simulink model "Q410_sim"  (R2021b)
settings: Solver=ode45  StartTime=0.0  StopTime=50  MinStep=0.0000001  RelTol=1e-3
values from neighbouring files (symbols this model uses):
  A = poly([-0.5 ,-3])    [Q410.m]
  A_m = [1 2*zeta*omega_n omega_n^2]    [Q410.m]
  alpha = .3    (= 0.3)    [Q410.m]
  B = 3    [Q410.m]
  P_0 = 1e12*eye(4)    [Q410.m]
  T = .0001    (= 0.0001)    [Q410.m]
settings Model: Creator=YSNsec  LastModifiedBy=YSNsec

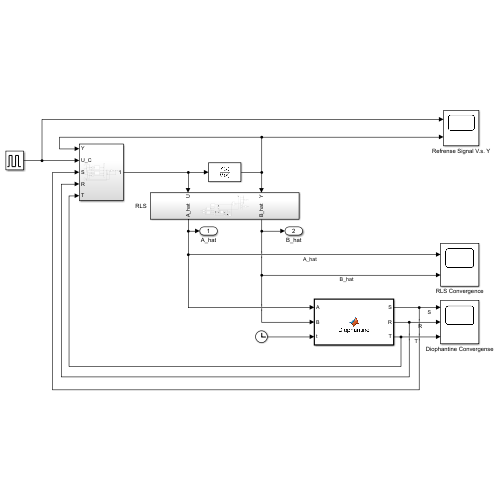
[thumbnail: Simulink's stored preview of the top-level diagram]
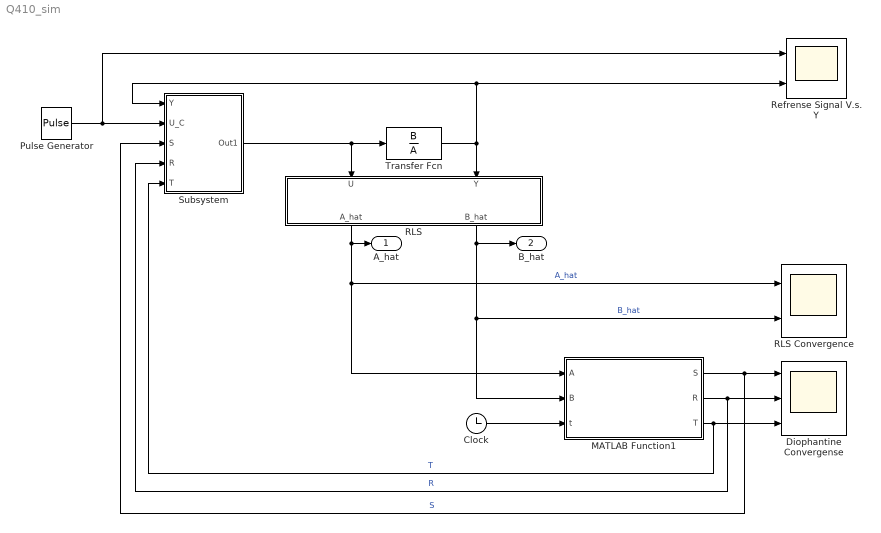
== system Q410_sim ==
  Clock : Clock
  Diophantine Convergense : Scope  NumInputPorts=3
  MATLAB Function1 : MATLAB Function  TreatAsAtomicUnit=on
  Pulse Generator : DiscretePulseGenerator  PulseType=Time based  Period=6  PulseWidth=50
  RLS : Subsystem
  RLS Convergence : Scope  NumInputPorts=2
  Refrense Signal V.s. Y : Scope  NumInputPorts=2
  Subsystem : Subsystem
  Transfer Fcn : TransferFcn  Numerator=B  Denominator=A
  A_hat : Outport  VectorParamsAs1DForOutWhenUnconnected=off
  B_hat : Outport  Port=2  VectorParamsAs1DForOutWhenUnconnected=off
  wires:
  Clock/1 -> MATLAB Function1/3(t)
  RLS/2(B_hat) -> B_hat/1, MATLAB Function1/2(B), RLS Convergence/2  "B_hat"
  RLS/1(A_hat) -> A_hat/1, RLS Convergence/1, MATLAB Function1/1(A)  "A_hat"
  MATLAB Function1/1(S) -> Diophantine Convergense/1, Subsystem/3(S)  "S"
  MATLAB Function1/2(R) -> Diophantine Convergense/2, Subsystem/4(R)  "R"
  MATLAB Function1/3(T) -> Diophantine Convergense/3, Subsystem/5(T)  "T"
  Transfer Fcn/1 -> Refrense Signal V.s. Y/2, Subsystem/1(Y), RLS/2(Y)
  Subsystem/1(Out1) -> Transfer Fcn/1, RLS/1(U)
  Pulse Generator/1 -> Subsystem/2(U_C), Refrense Signal V.s. Y/1

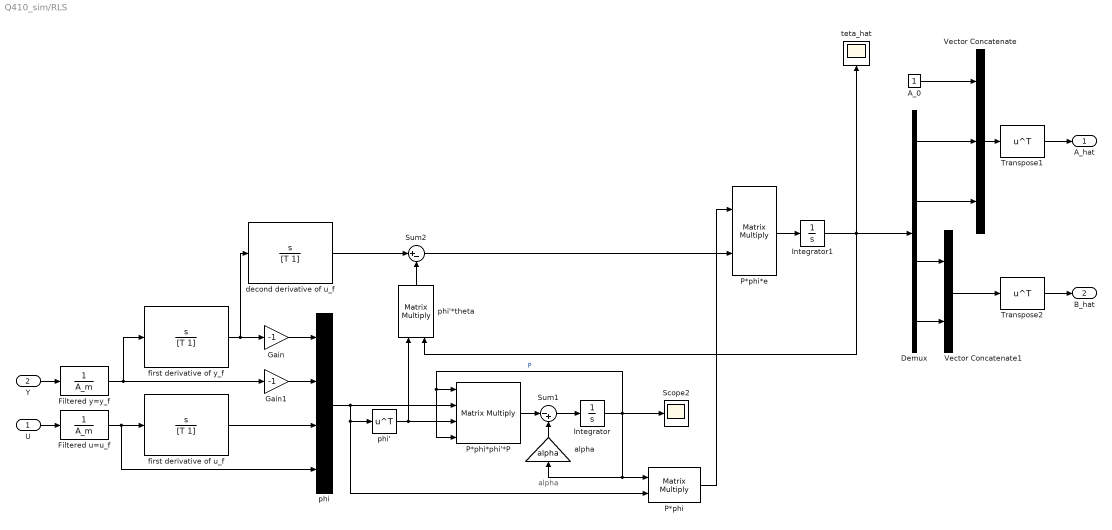
== system Q410_sim/RLS ==
  note: alpha
  U : Inport
  Y : Inport  Port=2
  A_0 : Constant
  Demux : Demux
  Filtered u=u_f : TransferFcn  Denominator=A_m
  Filtered y=y_f : TransferFcn  Denominator=A_m
  Gain : Gain  Gain=-1
  Gain1 : Gain  Gain=-1
  Integrator : Integrator  InitialCondition=P_0  LimitOutput=on
  Integrator1 : Integrator  InitialCondition=[0,0,0,0]  UpperSaturationLimit=100  LowerSaturationLimit=-100  ZeroCross=off
  P*phi : Product  Multiplication=Matrix(*)
  P*phi*e : Product  Multiplication=Matrix(*)
  P*phi*phi'*P : Product  Inputs=4  Multiplication=Matrix(*)
  Scope2 : Scope
  Sum1 : Sum  Inputs=|-+
  Sum2 : Sum  Inputs=|+-
  Transpose1 : Math  Operator=transpose  SignedPower=on  SaturateOnIntegerOverflow=on
  Transpose2 : Math  Operator=transpose  SignedPower=on  SaturateOnIntegerOverflow=on
  Vector Concatenate : Concatenate  NumInputs=3
  Vector Concatenate1 : Concatenate
  alpha : Gain  Gain=alpha
  decond derivative of u_f : TransferFcn  Numerator=[1 0]  Denominator=[T 1]
  first derivative of u_f : TransferFcn  Numerator=[1 0]  Denominator=[T 1]
  first derivative of y_f : TransferFcn  Numerator=[1 0]  Denominator=[T 1]
  phi : Concatenate  NumInputs=4
  phi' : Math  Operator=transpose  SignedPower=on  SaturateOnIntegerOverflow=on
  phi'*theta : Product  Multiplication=Matrix(*)
  "teta_hat " : Scope
  A_hat : Outport  VectorParamsAs1DForOutWhenUnconnected=off
  B_hat : Outport  Port=2  VectorParamsAs1DForOutWhenUnconnected=off
  wires:
  Demux/3 -> Vector Concatenate1/1
  Demux/1 -> Vector Concatenate/2
  Integrator/1 -> Scope2/1, P*phi*phi'*P/1, P*phi*phi'*P/4, P*phi/1, alpha/1  "P"
  phi'/1 -> phi'*theta/1, P*phi*phi'*P/3
  Integrator1/1 -> "teta_hat "/1, Demux/1, phi'*theta/2
  Gain1/1 -> phi/2
  Demux/4 -> Vector Concatenate1/2
  Demux/2 -> Vector Concatenate/3
  Transpose1/1 -> A_hat/1
  Sum1/1 -> Integrator/1
  P*phi*phi'*P/1 -> Sum1/1
  phi/1 -> P*phi/2, phi'/1, P*phi*phi'*P/2
  Vector Concatenate/1 -> Transpose1/1
  alpha/1 -> Sum1/2
  P*phi*e/1 -> Integrator1/1
  phi'*theta/1 -> Sum2/2
  Vector Concatenate1/1 -> Transpose2/1
  P*phi/1 -> P*phi*e/1
  Sum2/1 -> P*phi*e/2
  Gain/1 -> phi/1
  A_0/1 -> Vector Concatenate/1
  Transpose2/1 -> B_hat/1
  U/1 -> Filtered u=u_f/1
  Y/1 -> Filtered y=y_f/1
  first derivative of y_f/1 -> Gain/1, decond derivative of u_f/1
  decond derivative of u_f/1 -> Sum2/1
  Filtered y=y_f/1 -> Gain1/1, first derivative of y_f/1
  Filtered u=u_f/1 -> first derivative of u_f/1, phi/4
  first derivative of u_f/1 -> phi/3

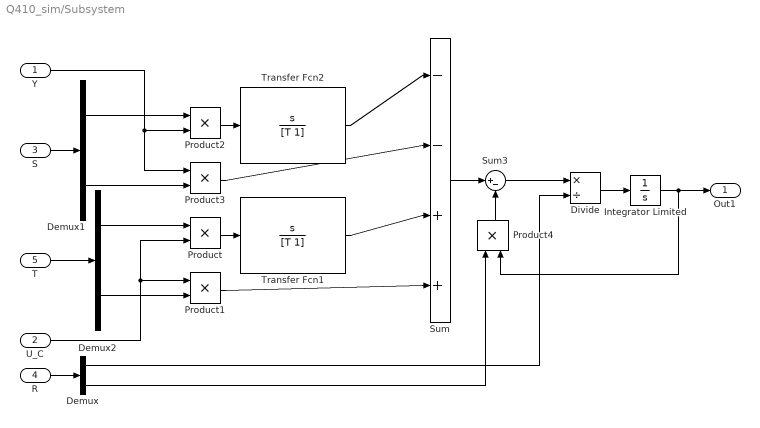
== system Q410_sim/Subsystem ==
  Y : Inport
  U_C : Inport  Port=2
  S : Inport  Port=3
  R : Inport  Port=4
  T : Inport  Port=5
  Demux : Demux  Outputs=2
  Demux1 : Demux  Outputs=2
  Demux2 : Demux  Outputs=2
  Divide : Product  Inputs=*/
  Integrator Limited : Integrator  LimitOutput=on  UpperSaturationLimit=1000  LowerSaturationLimit=-1000
  Product{,1..4} (5 alike) : Product
  Sum : Sum  Inputs=|--++
  Sum3 : Sum  Inputs=|+-
  Transfer Fcn1 : TransferFcn  Numerator=[1 0]  Denominator=[T 1]
  Transfer Fcn2 : TransferFcn  Numerator=[1 0]  Denominator=[T 1]
  Out1 : Outport
  wires:
  R/1 -> Demux/1
  Transfer Fcn2/1 -> Sum/1
  Product4/1 -> Sum3/2
  Product/1 -> Transfer Fcn1/1
  Product3/1 -> Sum/2
  Product1/1 -> Sum/4
  Transfer Fcn1/1 -> Sum/3
  Divide/1 -> Integrator Limited/1
  Sum3/1 -> Divide/1
  Product2/1 -> Transfer Fcn2/1
  Demux/2 -> Product4/1
  Sum/1 -> Sum3/1
  Demux/1 -> Divide/2
  Integrator Limited/1 -> Out1/1, Product4/2
  U_C/1 -> Product/2, Product1/1
  Demux1/1 -> Product2/1
  Demux1/2 -> Product3/2
  Y/1 -> Product3/1, Product2/2
  Demux2/1 -> Product/1
  Demux2/2 -> Product1/2
  T/1 -> Demux2/1
  S/1 -> Demux1/1

== matlab function Q410_sim/MATLAB Function1 ==
  data: S output; R output; A input; B input; T output; t input
function [ S, R ,T] = Diophantine(A,B,t )
if t>0.1
%% Calculating orders

omega_n=6;
zeta   =0.67;
A_m    =[1 2*zeta*omega_n omega_n^2];
A_o=[1 10];
A_c=conv(A_o,A_m);

alpha=conv(A_o,A_m);
d=1;
if(d<=0)
    disp('error, the delay d must be >=1')
end
na = length(A)-1;
nb = length(B)-1;
nr = nb + d - 1;
ns = na - 1;
nalpha = na + nb +d - 1;

%% initialization of M matrix and V matrix
M = zeros(nalpha, nalpha);
Y = zeros(nalpha, 1);
V = zeros(nalpha, 1);
Y(1:na, 1) = A(2:end);
V(1:nalpha, 1) = alpha(2:end);

%% M matrix filling
for i = 1: nalpha
    if(i<=nr)
        M(i:(length(A)+i-1), i) = A;
    else
        M(d+(i-(nr+1)):(d+(i-(nr+1)))+nb, i) = B;
    end
end

%% Solution of the Diophantine equation to find S, R polynomials 
theta = M\(V-Y);
R = [1; theta(1:nr)]';
S = theta((nr+1):end)';

T=A_o*A_m(end)/B(end);
else
R=[1,1];
S=[1,1];
T=[1,1];
end
